simulink model "problem3bilinear"  (R2020b)
settings: Solver=VariableStepAuto  StartTime=0.0  StopTime=10.0  RelTol=1e-3
settings Model: Creator=Shivashis  LastModifiedBy=Shivashis

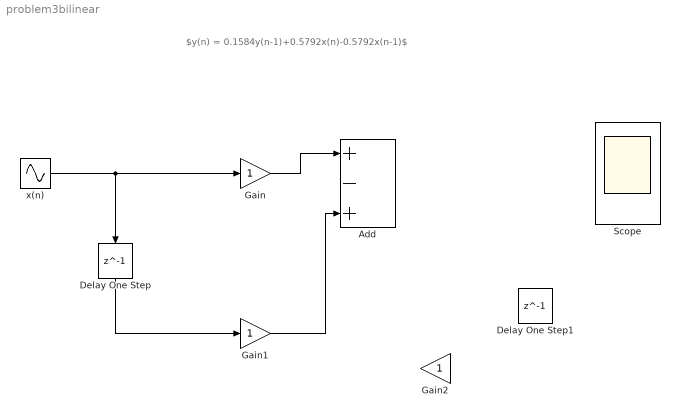
== system problem3bilinear ==
  note: $y(n) = 0.1584y(n-1)+0.5792x(n)-0.5792x(n-1)$
  Add : Sum  Inputs=+-+
  Delay One Step : Delay  DelayLength=1
  Delay One Step1 : Delay  DelayLength=1
  Gain : Gain
  Gain1 : Gain
  Gain2 : Gain
  Scope : Scope
  x(n) : Sin  Frequency=200  SampleTime=1/5000
  wires:
  x(n)/1 -> Delay One Step/1, Gain/1
  Gain/1 -> Add/1
  Delay One Step/1 -> Gain1/1
  Gain1/1 -> Add/3
